simulink model "receiver_from_dSPACE"  (R2018a)
settings: Solver=FixedStepDiscrete  StartTime=0.0  StopTime=inf  FixedStep=0.001  RelTol=1e-3  EnableMultiTasking=on
PostLoadFcn:
  | , if any(exist('dsrtsu_mdlpostloadfcn', 'file') == [2, 3, 6]), try dsrtsu_mdlpostloadfcn('Execute', bdroot); catch fprintf('Error in PostLoadFcn (dsrtsu_mdlpostloadfcn) for model "%s":\n %s\n', bdroot, lasterr); end, end,
undefined symbols (not defined in the file or in its folder): f
libraries: instrumentlib x1, dspnetwork x1
settings Model: DSRTSU_INTERNAL_RTI_VER=460  DSRTSU_INTERNAL_RTI_TYPE=rti1006  RTICANMMDATA=struct('GeneralSetupData',struct('modelroot','D:\StSoftware\Simulator_cabinTUD\Students\TestsPlatooning\programmas','generalsettings',struct('filesettings',struct('destfolder',struct('Name','RTICANMM_FILES','Check',1),'buildfolder',struct('Name','.','Check',1),'AbsDestfolder',struct('Name','D:\StSoftware\Simulator_cabinTUD\Students\TestsPlatooning\programmas\RTICANMM_FILES'),'AbsBuildfolder',struct('Name','D:\StSoftware\Simulator_cabinTUD\Students\TestsPlatooning\programmas'))),'options',struct('addpaths',1,'rmpaths',1,'addtrcexclusion',logical(1),'cannavigator',struct('checkmonitoring',0),'show_usrtrc',0,'use_usrtrc',0),'advanced',struct('options',[1 1 1 1 1 1 1 1 1 1 1 1 1 1 1 1 1 1 1 1 1 1 1 1 1 1 1 1 1 1 1 1 1 1 1 1 1 1 1 1 1 1 1 1 1 1 1 1 1 1 1 1 1 1 1 1 1 1 1 1 1 1 1 1 1 1 1 1 1 1 1 1 1 1 1 1 1 1 1 1 1 1 1 1 1 1 1 1 1 1 1 1 1 1 1 1 1 1 1 1]),'MPSetup',{{}},'modelname','receiver_SystemA','block','receiver_SystemA'))  DSRTSU_INTERNAL_RTIFPGA=50  Creator=Localadmin  LastModifiedBy=svenu
settings DataIOCC: LimitDataPoints=on  SaveFormat=Array
settings OptimizationCC: BlockReduction=off  OptimizeBlockIOStorage=off  BufferReuse=off  GlobalBufferReuse=off  ExpressionFolding=off  LocalBlockOutputs=off  LifeSpan=inf  OptimizeDataStoreBuffers=off  BusAssignmentInplaceUpdate=off
settings DebuggingCC: SolverPrmCheckMsg=warning  ParameterPrecisionLossMsg=none  SFUnexpectedBacktrackingDiag=warning  SFNoUnconditionalDefaultTransitionDiag=warning  SFExecutionAtInitializationDiag=none
settings HardwareCC: ProdBitPerPointer=32  ProdBitPerSizeT=32  ProdBitPerPtrDiffT=32  ProdLargestAtomicFloat=None  ProdWordSize=32  ProdHWDeviceType=Generic->Custom  TargetIntDivRoundTo=Zero  TargetEndianess=LittleEndian  TargetHWDeviceType=Generic->Custom
settings ModelReferenceCC: PropagateSignalLabelsOutOfModel=off
settings RTWCC: SystemTargetFile=rti1006.tlc  MakeCommand=make_rti  TemplateMakefile=rti1006.tmf  Description=dSPACE DS1006 Hardware Platform
settings CodeAppCC: StateflowObjectComments=on
settings STFCustomTargetCC: ParMdlRefBuildCompliant=on  GeneratePreprocessorConditionals=Disable all  MatFileLogging=on  SystemTargetFile=rti1006.tlc
settings GRTTargetCC: TargetLangStandard=C89/C90 (ANSI)  CompOptLevelCompliant=off  ConcurrentExecutionCompliant=off  GeneratePreprocessorConditionals=Disable all  CombineOutputUpdateFcns=off  CPPClassGenCompliant=off  GRTInterface=on  UseToolchainInfoCompliant=off  ExtModeMexFile=noextcomm
settings ConfigComp: CovMetricSettings=dw  CovHtmlReporting=on  CovSaveCumulativeToWorkspaceVar=on  CovSaveSingleToWorkspaceVar=on  CovExternalEMLEnable=off  CovSFcnEnable=off

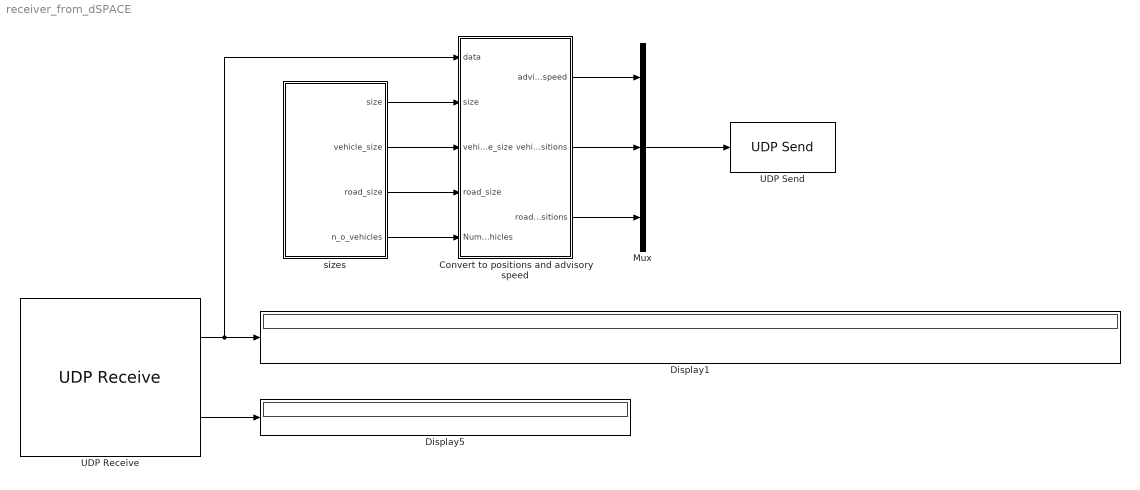
== system receiver_from_dSPACE ==
  Convert to positions and advisory speed : Subsystem
  Display1 : Display
  Display5 : Display
  Mux : Mux  Inputs=3
  UDP Receive : instrumentlib/UDP Receive  Host=127.0.0.1  Port=50055  LocalPort=50055  EnablePortSharing=off  GetLatestData=off  DataSize=30  DataType=single  ASCIIFormatting=%f,  Terminator=LF  ByteOrder=BigEndian  EnableBlockingMode=off  Timeout=10  SampleTime=10  LocalAddress=0.0.0.0
      settings: SourceProductName=Instrument Control Toolbox
  UDP Send : dspnetwork/UDP Send  remoteURL='127.0.0.1'  remotePort=11000  localURL='0.0.0.0'  localPortSource=Automatically determine  localPort=-1  sampletime=-1  blockPlatform=[]  separateLengthPort=0
      settings: SourceProductName=DSP System Toolbox  SourceProductBaseCode=DS
  sizes : Subsystem
  wires:
  UDP Receive/2 -> Display5/1
  UDP Receive/1 -> Convert to positions and advisory speed/1(data), Display1/1
  sizes/3(road_size) -> Convert to positions and advisory speed/4(road_size)
  sizes/1(size) -> Convert to positions and advisory speed/2(size)
  sizes/2(vehicle_size) -> Convert to positions and advisory speed/3(vehicle_size)
  Convert to positions and advisory speed/1(advisory_speed) -> Mux/1
  Convert to positions and advisory speed/2(vehicle_positions) -> Mux/2
  Convert to positions and advisory speed/3(road_positions) -> Mux/3
  Mux/1 -> UDP Send/1
  sizes/4(n_o_vehicles) -> Convert to positions and advisory speed/5(Number of vehicles)

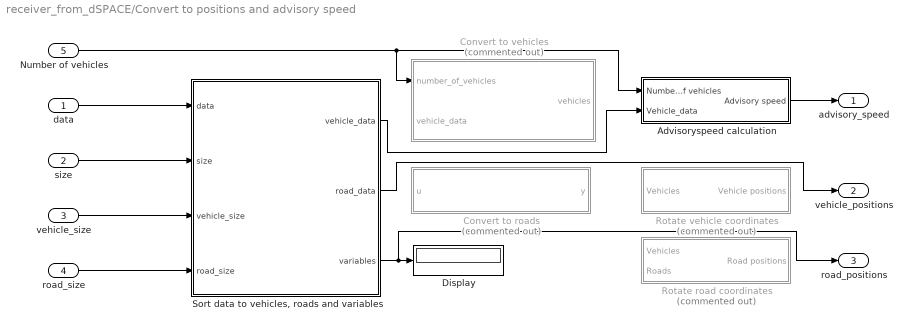
== system receiver_from_dSPACE/Convert to positions and advisory speed ==
  data : Inport
  size : Inport  Port=2
  vehicle_size : Inport  Port=3
  road_size : Inport  Port=4
  Number of vehicles : Inport  Port=5
  Advisoryspeed calculation : Subsystem
  Convert to roads : MATLAB Function  Commented=on  TreatAsAtomicUnit=on
  Convert to vehicles : MATLAB Function  Commented=on  TreatAsAtomicUnit=on
  Display : Display
  Rotate road coordinates : Subsystem  Commented=on
  Rotate vehicle coordinates : Subsystem  Commented=on
  "Sort data to vehicles, roads and variables" : MATLAB Function  TreatAsAtomicUnit=on
  advisory_speed : Outport
  vehicle_positions : Outport  Port=2
  road_positions : Outport  Port=3
  wires:
  data/1 -> "Sort data to vehicles, roads and variables"/1(data)
  size/1 -> "Sort data to vehicles, roads and variables"/2(size)
  vehicle_size/1 -> "Sort data to vehicles, roads and variables"/3(vehicle_size)
  road_size/1 -> "Sort data to vehicles, roads and variables"/4(road_size)
  Advisoryspeed calculation/1(Advisory speed) -> advisory_speed/1
  "Sort data to vehicles, roads and variables"/3(variables) -> road_positions/1, Display/1
  "Sort data to vehicles, roads and variables"/2(road_data) -> vehicle_positions/1
  "Sort data to vehicles, roads and variables"/1(vehicle_data) -> Advisoryspeed calculation/2(Vehicle_data)
  Number of vehicles/1 -> Advisoryspeed calculation/1(Number of vehicles), Convert to vehicles/1(number_of_vehicles)

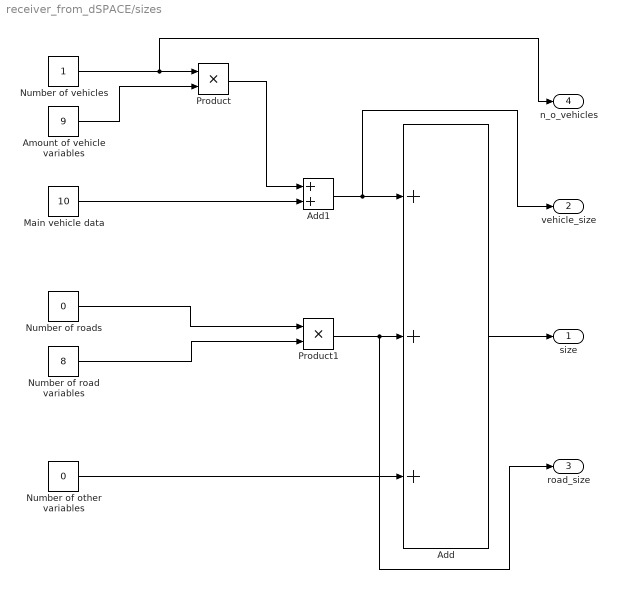
== system receiver_from_dSPACE/sizes ==
  Add : Sum  Inputs=+++
  Add1 : Sum
  Amount of vehicle variables : Constant  Value=9
  Main vehicle data : Constant  Value=10
  Number of other variables : Constant  Value=0
  Number of road variables : Constant  Value=8
  Number of roads : Constant  Value=0
  Number of vehicles : Constant
  Product : Product
  Product1 : Product
  size : Outport
  vehicle_size : Outport  Port=2
  road_size : Outport  Port=3
  n_o_vehicles : Outport  Port=4
  wires:
  Number of other variables/1 -> Add/3
  Number of road variables/1 -> Product1/2
  Number of roads/1 -> Product1/1
  Number of vehicles/1 -> n_o_vehicles/1, Product/1
  Product1/1 -> road_size/1, Add/2
  Add/1 -> size/1
  Amount of vehicle variables/1 -> Product/2
  Product/1 -> Add1/1
  Add1/1 -> vehicle_size/1, Add/1
  Main vehicle data/1 -> Add1/2

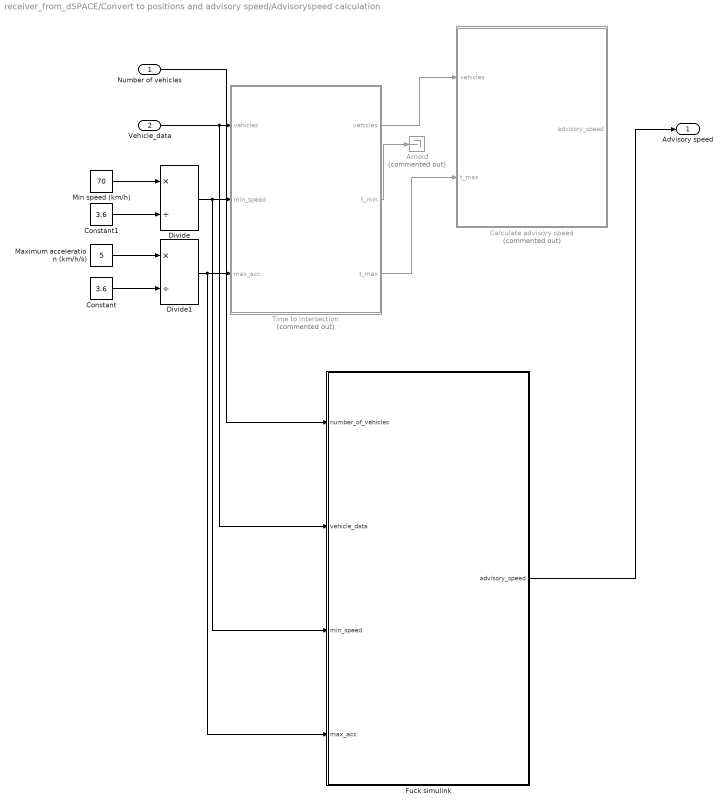
== system receiver_from_dSPACE/Convert to positions and advisory speed/Advisoryspeed calculation ==
  Number of vehicles : Inport
  Vehicle_data : Inport  Port=2
  Arnold : Terminator  Commented=on
  Calculate advisory speed : MATLAB Function  Commented=on  TreatAsAtomicUnit=on
  Constant : Constant  Value=3.6
  Constant1 : Constant  Value=3.6
  Divide : Product  Inputs=*/
  Divide1 : Product  Inputs=*/
  Fuck simulink : MATLAB Function  TreatAsAtomicUnit=on
  Maximum acceleration (km/h/s) : Constant  Value=5
  Min speed (km/h) : Constant  Value=70
  Time to intersection : MATLAB Function  Commented=on  TreatAsAtomicUnit=on
  Advisory speed : Outport
  wires:
  Vehicle_data/1 -> Fuck simulink/2(vehicle_data), Time to intersection/1("vehicles ")
  Min speed (km/h)/1 -> Divide/1
  Maximum acceleration (km/h/s)/1 -> Divide1/1
  Time to intersection/3(t_max) -> Calculate advisory speed/2(t_max)
  Constant1/1 -> Divide/2
  Constant/1 -> Divide1/2
  Divide1/1 -> Fuck simulink/4(max_acc), Time to intersection/3(max_acc)
  Time to intersection/2(t_min) -> Arnold/1
  Divide/1 -> Fuck simulink/3(min_speed), Time to intersection/2(min_speed)
  Time to intersection/1(vehicles) -> Calculate advisory speed/1(vehicles)
  Number of vehicles/1 -> Fuck simulink/1(number_of_vehicles)
  Fuck simulink/1(advisory_speed) -> Advisory speed/1

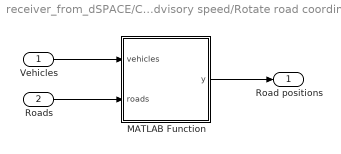
== system receiver_from_dSPACE/Convert to positions and advisory speed/Rotate road coordinates ==
  Vehicles : Inport
  Roads : Inport  Port=2
  MATLAB Function : MATLAB Function  TreatAsAtomicUnit=on
  Road positions : Outport
  wires:
  Vehicles/1 -> MATLAB Function/1(vehicles)
  Roads/1 -> MATLAB Function/2(roads)
  MATLAB Function/1(y) -> Road positions/1

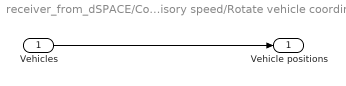
== system receiver_from_dSPACE/Convert to positions and advisory speed/Rotate vehicle coordinates ==
  Vehicles : Inport
  Vehicle positions : Outport
  wires:
  Vehicles/1 -> Vehicle positions/1

== matlab function receiver_from_dSPACE/Convert to positions and advisory speed/Convert to vehicles ==
  data: number_of_vehicles input; vehicle_data input; vehicles output
function vehicles = vehicle_convert(number_of_vehicles, vehicle_data)
    vehicles = cell(number_of_vehicles, 1);
    
    % Define main vehicle
    current_vehicle = vehicle_data(1:10);
        
    part_nr = current_vehicle(1);
    type = [current_vehicle(2), current_vehicle(3)];
    position = [current_vehicle(4), current_vehicle(5), current_vehicle(6)];
    dynamics = [current_vehicle(7), current_vehicle(8), current_vehicle(9), current_vehicle(10)];
    
    vehicles{1} = [part_nr, type, position, dynamics];
    
    % Define other vehicles
    index = 2;
    for i = 11:9:length(vehicle_data)
        current_vehicle = vehicle_data(i:i+8);
        
        part_nr = current_vehicle(1);
        type = [current_vehicle(2), current_vehicle(3)];
        position = [current_vehicle(4), current_vehicle(5), current_vehicle(6)];
        dynamics = [current_vehicle(7), current_vehicle(8), current_vehicle(9)];
    
        vehicles{index} = [part_nr, type, position, dynamics];
        index = index + 1;
    end
end

== matlab function receiver_from_dSPACE/Convert to positions and advisory speed/Sort data to vehicles, roads and variables ==
  data: data input; vehicle_data output; road_data output; size input; vehicle_size input; road_size input; variables output
function [vehicle_data, road_data, variables] = sort(data, size, vehicle_size, road_size)
    vehicle_data = 0;
    road_data = 0;
    variables = 0;
    
    if vehicle_size > 0
        vehicle_data = data(1:vehicle_size);
        if road_size > 0
            road_data = data(vehicle_size + 1: vehicle_size + road_size + 1);
            variables = data(vehicle_size + road_size + 2: size);
        end
    end
end

== matlab function receiver_from_dSPACE/Convert to positions and advisory speed/Advisoryspeed calculation/Time to intersection ==
  data: vehicles output; t_min output; vehicles input; min_speed input; max_acc input; t_max output
function [vehicles, t_min, t_max] = calculate_time_to_intersection(vehicles, min_speed, max_acc)
    
%% Calculate time t_min to intersection with minimum speed 
    % t_min = 2 * vehicle.Dynamics.DisToInter / (min_speed + vehicle.Dynamics.Velocity
    t_min = 2 * vehicles{1, 1}(8) / (min_speed + vehicles{1, 1}(7));
    
%% Calculate time t_max to intersection with maximum acceleration
    % t_max = max(roots[max_acc/2, vehicle.Dynamics.Velocity,
    % -vehicle.Dynamics.DisToInter]))
    t_max = max(roots([max_acc/2, vehicles{1, 1}(7), -vehicles{1, 1}(8)]));
    
%% Calculate predicted time to intersection
    vehicles{1, 2} = zeros(1,3);
    % vehicle.TimeToInter = max(roots([vehicle.Dynamics.Acc/2,
    % vehicle.Dynamics.Velocity, -vehicle.Dynamics.DisToInter]))
    vehicles{1, 2}(1) = max(roots([vehicles{1, 1}(10)/2, vehicles{1, 1}(7), -vehicles{1, 1}(8)]));
    % speed_at_inter = vehicle.Dynamics.Velocity + vehicle.Dynamics.Acc * vehicle.TimeToInter;
    speed_at_inter = vehicles{1, 1}(7) + vehicles{1, 1}(10) * vehicles{1, 2}(1);
    % vehicle.TimeToInterFront = vehicle.TimeToInter - vehicle.Type.CarLength / speed_at_inter;
    vehicles{1, 2}(2) = vehicles{1, 2}(1) - vehicles{1, 1}(3) / speed_at_inter;
    % vehicle.TimeToInterBack = vehicle.TimeToInter + vehicle.Type.CarLength / speed_at_inter;
    vehicles{1, 2}(3) = vehicles{1, 2}(1) + vehicles{1, 1}(3) / speed_at_inter;
end

== matlab function receiver_from_dSPACE/Convert to positions and advisory speed/Advisoryspeed calculation/Calculate advisory speed ==
  data: vehicles input; advisory_speed output; t_max input
function advisory_speed = calculate_advisory_speed(vehicles, t_max)

%% Devide client from HMI and other vehicles
    main_vehicle = vehicles(1);
    vehicles = vehicles(2:end);
    
%% Calculate time to reach intersection for other vehicles for front, middle and back
    for i = 1:length(vehicles)
        vehicle = vehicles(i);
        vehicle.TimeToInter = vehicle.Dynamics.DisToInter / vehicle.Dynamics.Velocity;
        vehicle.TimeToInterFront = (vehicle.Dynamics.DisToInter - vehicle.Type.CarLength / 2) / vehicle.Dynamics.Velocity;
        vehicle.TimeToInterBack = (vehicle.Dynamics.DisToInter + vehicle.Type.CarLength / 2) / vehicle.Dynamics.Velocity;
    end
    
%% Sort vehicles on time to inter in order from long to short
    [~, ind] = sort([vehicles.TimeToInter]);
    vehicles = fliplr(vehicles(ind));
    
%% Delete vehicles which are not in the right lane
    index_to_delete = [];
    for i = 1:length(vehicles)
        if vehicles(i).Dynamics.Lane ~= 0
            index_to_delete = [index_to_delete, i];
        end
    end
    vehicles(index_to_delete) = [];
    
%% Create an array with gaps

    % Define begin- and endtime of section and whether it is a gap or not
    gaps = Gaps.empty(1,0)';
    
    % Define first no_gap
    gaps(1) = Gap(vehicle(1).TimeToInterBack, vehicle(1).TimeToInterFront, false);
    
    for i = 2:length(vehicles)
        gap = Gap(vehicle(i-1).TimeToInterFront, vehicle(i).TimeToInterBack, true);
        no_gap = Gap(vehicle(i).TimeToInterBack, vehicle(i).TimeToInterFront, false);
        gaps = [gaps, gap, no_gap];
    end
    
    if vehicles(end).TimeToInterFront > t_max
        gap = Gap(vehicles(end).TimeToInterFront, t_max, true);
        gaps = [gaps, gap];
    end
    
%% Decide which gap is the best gap
    % Sort gaps on time from predicted time
    begin_times = gaps.BeginTime;
    end_times = gaps.EndTime;
    time = (begin_times + end_times) / 2 - main_vehicle.TimeToInter;
    [~, ind] = sort(time);
    gaps = gaps(ind);
    
    % Find the nearest gap with an optimal size
    target_gap = find_target_gap(gaps);
    
    % Calculate desired speed at intersection
    advisory_speed = 2 * main_vehicle.Dynamics.DisToInter / target_gap.get_time_to_inter() + main_vehicle.Dynamics.Velocity; 
    
    % Round to 5
    advisory_speed = round(advisory_speed / 5) * 5;
end

== matlab function receiver_from_dSPACE/Convert to positions and advisory speed/Convert to roads ==
  data: u input; y output
function y = fcn(u)
%TODO
y = u;

== matlab function receiver_from_dSPACE/Convert to positions and advisory speed/Rotate road coordinates/MATLAB Function ==
  data: vehicles input; y output; roads input
function y = fcn(vehicles, roads)

y = 1;

== matlab function receiver_from_dSPACE/Convert to positions and advisory speed/Advisoryspeed calculation/Fuck simulink ==
  data: number_of_vehicles input; advisory_speed output; vehicle_data input; min_speed input; max_acc input
function advisory_speed = calculate_advisory_speed_part_fuck_simulink(number_of_vehicles, vehicle_data, min_speed, max_acc)
    vehicles = vehicle_convert(number_of_vehicles, vehicle_data);
    [vehicles, t_min, t_max] = calculate_time_to_intersection(vehicles, min_speed, max_acc);
    advisory_speed = calculate_advisory_speed(vehicles, t_max);
end
